simulink model "halfcarbody_tb"  (R2024b)
settings: Solver=VariableStepAuto  StartTime=0.0  StopTime=10.0  RelTol=1e-3
settings Model: Creator=sebam  LastModifiedBy=sebam

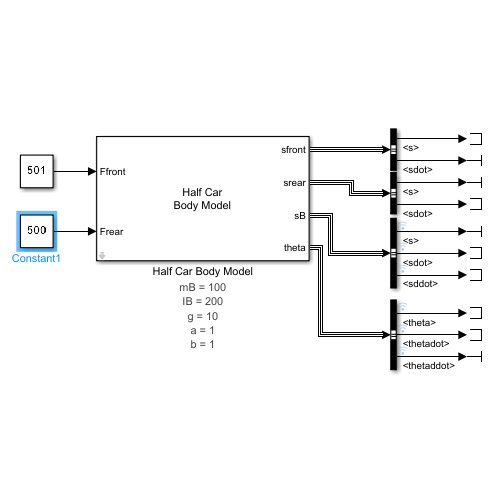
[thumbnail: Simulink's stored preview of the top-level diagram]
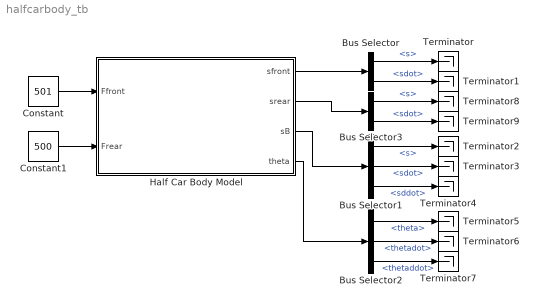
== system halfcarbody_tb ==
  Bus Selector : BusSelector  OutputSignals=s,sdot
  Bus Selector1 : BusSelector  OutputSignals=s,sdot,sddot
  Bus Selector2 : BusSelector  OutputSignals=theta,thetadot,thetaddot
  Bus Selector3 : BusSelector  OutputSignals=s,sdot
  Constant : Constant  Value=501
  Constant1 : Constant  Value=500
  Half Car Body Model : Subsystem  mask{mB=100, IB=200, g=10, a=1, b=1}
      mask prompts: mB "Mass (mB)"; IB "Moment of Inertia (IB)"; g "Gravity (g)"; a "Length A (a)"; b "Length B (b)"
      settings: AttributesFormatString=|
      | mB = %<mB>
      | IB = %<IB>
      | g = %<g>
      | a = %<a>
      | b = %<b>
      mask Display: fprintf("Half Car\nBody Model")
  Terminator{,1..9} (10 alike) : Terminator
  wires:
  Constant/1 -> Half Car Body Model/1(Ffront)
  Constant1/1 -> Half Car Body Model/2(Frear)
  Half Car Body Model/1(sfront) -> Bus Selector/1
  Bus Selector/1 -> Terminator/1  "<s>"
  Bus Selector/2 -> Terminator1/1  "<sdot>"
  Half Car Body Model/3(sB) -> Bus Selector1/1
  Bus Selector1/1 -> Terminator2/1  "<s>"
  Bus Selector1/2 -> Terminator3/1  "<sdot>"
  Bus Selector1/3 -> Terminator4/1  "<sddot>"
  Half Car Body Model/4(theta) -> Bus Selector2/1
  Bus Selector2/1 -> Terminator5/1  "<theta>"
  Bus Selector2/2 -> Terminator6/1  "<thetadot>"
  Bus Selector2/3 -> Terminator7/1  "<thetaddot>"
  Half Car Body Model/2(srear) -> Bus Selector3/1
  Bus Selector3/1 -> Terminator8/1  "<s>"
  Bus Selector3/2 -> Terminator9/1  "<sdot>"

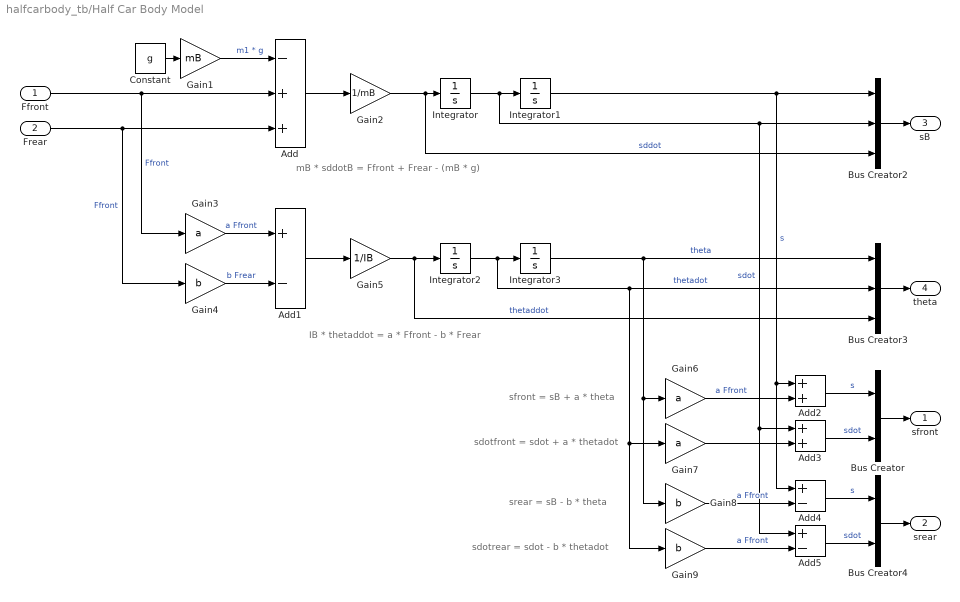
== system halfcarbody_tb/Half Car Body Model ==
  note: sfront = sB + a * theta
  note: IB * thetaddot = a * Ffront - b * Frear
  note: mB * sddotB = Ffront + Frear - (mB * g)
  note: sdotfront = sdot + a * thetadot
  note: srear = sB - b * theta
  note: sdotrear = sdot - b * thetadot
  Ffront : Inport
  Frear : Inport  Port=2
  Add : Sum  Inputs=-++
  Add1 : Sum  Inputs=+-
  Add2 : Sum
  Add3 : Sum
  Add4 : Sum  Inputs=+-
  Add5 : Sum  Inputs=+-
  Bus Creator : BusCreator  Inputs=2
  Bus Creator2 : BusCreator  Inputs=3
  Bus Creator3 : BusCreator  Inputs=3
  Bus Creator4 : BusCreator  Inputs=2
  Constant : Constant  Value=g
  Gain1 : Gain  Gain=mB
  Gain2 : Gain  Gain=1/mB
  Gain3 : Gain  Gain=a
  Gain4 : Gain  Gain=b
  Gain5 : Gain  Gain=1/IB
  Gain6 : Gain  Gain=a
  Gain7 : Gain  Gain=a
  Gain8 : Gain  Gain=b
  Gain9 : Gain  Gain=b
  Integrator{,1..3} (4 alike) : Integrator
  sfront : Outport
  srear : Outport  Port=2
  sB : Outport  Port=3
  theta : Outport  Port=4
  wires:
  Integrator1/1 -> Add4/1, Add2/1, Bus Creator2/1  "s"
  Add/1 -> Gain2/1
  Constant/1 -> Gain1/1
  Gain1/1 -> Add/1  "m1 * g"
  Gain2/1 -> Bus Creator2/3, Integrator/1  "sddot"
  Bus Creator/1 -> sfront/1
  Bus Creator4/1 -> srear/1
  Bus Creator2/1 -> sB/1
  Integrator/1 -> Integrator1/1, Add5/1, Add3/1, Bus Creator2/2  "sdot"
  Add3/1 -> Bus Creator/2  "sdot"
  Gain3/1 -> Add1/1  "a Ffront"
  Gain4/1 -> Add1/2  "b Frear"
  Add1/1 -> Gain5/1
  Gain5/1 -> Bus Creator3/3, Integrator2/1  "thetaddot"
  Integrator2/1 -> Gain9/1, Gain7/1, Bus Creator3/2, Integrator3/1  "thetadot"
  Integrator3/1 -> Gain8/1, Gain6/1, Bus Creator3/1  "theta"
  Bus Creator3/1 -> theta/1
  Add2/1 -> Bus Creator/1  "s"
  Gain6/1 -> Add2/2  "a Ffront"
  Gain7/1 -> Add3/2
  Add4/1 -> Bus Creator4/1  "s"
  Add5/1 -> Bus Creator4/2  "sdot"
  Gain8/1 -> Add4/2  "a Ffront"
  Gain9/1 -> Add5/2  "a Ffront"
  Ffront/1 -> Gain3/1, Add/2  "Ffront"
  Frear/1 -> Gain4/1, Add/3  "Ffront"
